simulink model "ibob_phased_array_2k"  (Simulink 7.1)
settings: Solver=ode45  StartTime=0.0  StopTime=70  RelTol=1e-3
undefined symbols (not defined in the file or in its folder): iBOB
libraries: xbsIndex_r4 x1407, xps_library x46, cfa_library x16, casper_library_sources x8, casper_library_misc x4
(part 3 of 18)

== system ibob_phased_array_2k/gain_calib3 ==
  gain : Inport  OutDataType=sfix(16)  OutScaling=2^0
  in : Inport  Port=2  OutDataType=sfix(16)  OutScaling=2^0
  Concat : xbsIndex_r4/Concat  num_inputs=4  dbl_ovrd=off  block_type=concat
      settings: block_version=10.1.3
  Delay{1..4} (4 alike) : xbsIndex_r4/Delay  en=off  latency=1  dbl_ovrd=off  reg_retiming=off  block_type=delay
  Mult{,1..3} (4 alike) : xbsIndex_r4/Mult  precision=Full  arith_type="Signed  (2's comp)"  n_bits=8  bin_pt=2  quantization=Truncate  overflow=Wrap  en=off  latency=7  dbl_ovrd=off  use_behavioral_HDL=off  use_embedded=on  opt=Speed  optimum_pipeline=off  pipeline=on  use_rpm=on  placement_style=Rectangular shape  block_type=mult
      settings: infoedit=Hardware notes: To use the internal pipeline stage of the dedicated multiplier you must select 'Pipeline for maximum performance'.  xl_area=[0, 0, 0, 0, 0, 0, 0]  block_version=10.1.3
  Reinterpret{,1..3} (4 alike) : xbsIndex_r4/Reinterpret  force_arith_type=on  arith_type=Unsigned  force_bin_pt=on  bin_pt=0  block_type=reinterpret
      settings: infoedit="Changes signal type without altering the binary representation.   You can changed the signal between signed and unsigned, and relocate the binary point.<P><P>Hardware notes: In hardware this block costs nothing.<P><P>Example:  Suppose the input is 6 bits wide, signed, with 2 fractional bits, and the output is forced to unsigned with 0 fractional bits.  Then an input of -2.0 (1110.00 in binary 2's complement) becomes an output of 56 (111000 in binary)."  block_version=10.1.3
  Reinterpret4 : xbsIndex_r4/Reinterpret  force_arith_type=on  arith_type=Unsigned  force_bin_pt=on  bin_pt=7  block_type=reinterpret
      settings: infoedit="Changes signal type without altering the binary representation.   You can changed the signal between signed and unsigned, and relocate the binary point.<P><P>Hardware notes: In hardware this block costs nothing.<P><P>Example:  Suppose the input is 6 bits wide, signed, with 2 fractional bits, and the output is forced to unsigned with 0 fractional bits.  Then an input of -2.0 (1110.00 in binary 2's complement) becomes an output of 56 (111000 in binary)."  block_version=10.1.3
  Slice2 : xbsIndex_r4/Slice  nbits=8  boolean_output=off  mode=Lower Bit Location + Width  bit1=0  base1=MSB of Input  bit0=0  base0=LSB of Input  dbl_ovrd=off  block_type=slice
      settings: infoedit="Extracts a given range of bits from each input sample and presents it at the output.  The output type is ordinarily unsigned with binary point at zero, but can be Boolean when the slice is one bit wide.<P><P>Hardware notes: In hardware this block costs nothing."  block_version=10.1.3
  convert1 : Subsystem  AncestorBlock=casper_library_misc/convert  mask(convert){bin_pt_in=7, n_bits_out=8, bin_pt_out=0, quantization=Round  (unbiased: +/- Inf), overflow=Saturate, latency=1}
      mask prompts: bin_pt_in "Binary Point In"; n_bits_out "Bit Width Out"; bin_pt_out "Binary Point Out"
      mask help:
      | Convert input value to the specified bit width and precision.
      |
      | Does not support upscaling number of fractional bits (eg 8_5 to 8_4 is ok, but not 8_4 to 8_5).
      mask init: same as ibob_phased_array_2k/gain_calib0/convert1
      settings: AttributesFormatString=|
      | N_7 ==> 8_0
      | round inf, saturate
      | latency = 1
      mask Help:
      | <pre>
      | Description::
      | 
      | Outputs converted version of the input.
      | 
      | Mask Parameters::
      | 
      | Binary Point In (bin_pt_in): Specifies the binary point location in the input.
      | 
      | Bit Width Out (n_bits_out): Specifies the width of the output.
      | 
      | Binary Point Out (bin_pt_out): Specifies the binary point location in the output.
      | 
      | Quantization (quantization): Specifies quantization handling.
      | 
      | Overflow (overflow): Specifies overflow handling.
      | 
      | Latency (latency): Specifies the latency of the underlying adder block, which is the overall
      | latency of this block as well.
      | </pre>
      mask StyleString: edit,edit,edit,popup(Truncate|Round  (unbiased: +/- Inf)|Round  (unbiased: Even Values)|Round  (unbiased: Zero)|Round  (unbiased: Odd Values)|Round  (biased: Up)|Round  (biased: Down)),popup(Wrap|Saturate|Error),edit
  convert2 : Subsystem  AncestorBlock=casper_library_misc/convert  mask(convert){bin_pt_in=7, n_bits_out=8, bin_pt_out=0, quantization=Round  (unbiased: +/- Inf), overflow=Saturate, latency=1}
      mask prompts: bin_pt_in "Binary Point In"; n_bits_out "Bit Width Out"; bin_pt_out "Binary Point Out"
      mask help:
      | Convert input value to the specified bit width and precision.
      |
      | Does not support upscaling number of fractional bits (eg 8_5 to 8_4 is ok, but not 8_4 to 8_5).
      mask init: same as ibob_phased_array_2k/gain_calib0/convert1
      settings: AttributesFormatString=|
      | N_7 ==> 8_0
      | round inf, saturate
      | latency = 1
      mask Help:
      | <pre>
      | Description::
      | 
      | Outputs converted version of the input.
      | 
      | Mask Parameters::
      | 
      | Binary Point In (bin_pt_in): Specifies the binary point location in the input.
      | 
      | Bit Width Out (n_bits_out): Specifies the width of the output.
      | 
      | Binary Point Out (bin_pt_out): Specifies the binary point location in the output.
      | 
      | Quantization (quantization): Specifies quantization handling.
      | 
      | Overflow (overflow): Specifies overflow handling.
      | 
      | Latency (latency): Specifies the latency of the underlying adder block, which is the overall
      | latency of this block as well.
      | </pre>
      mask StyleString: edit,edit,edit,popup(Truncate|Round  (unbiased: +/- Inf)|Round  (unbiased: Even Values)|Round  (unbiased: Zero)|Round  (unbiased: Odd Values)|Round  (biased: Up)|Round  (biased: Down)),popup(Wrap|Saturate|Error),edit
  convert3 : Subsystem  AncestorBlock=casper_library_misc/convert  mask(convert){bin_pt_in=7, n_bits_out=8, bin_pt_out=0, quantization=Round  (unbiased: +/- Inf), overflow=Saturate, latency=1}
      mask prompts: bin_pt_in "Binary Point In"; n_bits_out "Bit Width Out"; bin_pt_out "Binary Point Out"
      mask help:
      | Convert input value to the specified bit width and precision.
      |
      | Does not support upscaling number of fractional bits (eg 8_5 to 8_4 is ok, but not 8_4 to 8_5).
      mask init: same as ibob_phased_array_2k/gain_calib0/convert1
      settings: AttributesFormatString=|
      | N_7 ==> 8_0
      | round inf, saturate
      | latency = 1
      mask Help:
      | <pre>
      | Description::
      | 
      | Outputs converted version of the input.
      | 
      | Mask Parameters::
      | 
      | Binary Point In (bin_pt_in): Specifies the binary point location in the input.
      | 
      | Bit Width Out (n_bits_out): Specifies the width of the output.
      | 
      | Binary Point Out (bin_pt_out): Specifies the binary point location in the output.
      | 
      | Quantization (quantization): Specifies quantization handling.
      | 
      | Overflow (overflow): Specifies overflow handling.
      | 
      | Latency (latency): Specifies the latency of the underlying adder block, which is the overall
      | latency of this block as well.
      | </pre>
      mask StyleString: edit,edit,edit,popup(Truncate|Round  (unbiased: +/- Inf)|Round  (unbiased: Even Values)|Round  (unbiased: Zero)|Round  (unbiased: Odd Values)|Round  (biased: Up)|Round  (biased: Down)),popup(Wrap|Saturate|Error),edit
  convert4 : Subsystem  AncestorBlock=casper_library_misc/convert  mask(convert){bin_pt_in=7, n_bits_out=8, bin_pt_out=0, quantization=Round  (unbiased: +/- Inf), overflow=Saturate, latency=1}
      mask prompts: bin_pt_in "Binary Point In"; n_bits_out "Bit Width Out"; bin_pt_out "Binary Point Out"
      mask help:
      | Convert input value to the specified bit width and precision.
      |
      | Does not support upscaling number of fractional bits (eg 8_5 to 8_4 is ok, but not 8_4 to 8_5).
      mask init: same as ibob_phased_array_2k/gain_calib0/convert1
      settings: AttributesFormatString=|
      | N_7 ==> 8_0
      | round inf, saturate
      | latency = 1
      mask Help:
      | <pre>
      | Description::
      | 
      | Outputs converted version of the input.
      | 
      | Mask Parameters::
      | 
      | Binary Point In (bin_pt_in): Specifies the binary point location in the input.
      | 
      | Bit Width Out (n_bits_out): Specifies the width of the output.
      | 
      | Binary Point Out (bin_pt_out): Specifies the binary point location in the output.
      | 
      | Quantization (quantization): Specifies quantization handling.
      | 
      | Overflow (overflow): Specifies overflow handling.
      | 
      | Latency (latency): Specifies the latency of the underlying adder block, which is the overall
      | latency of this block as well.
      | </pre>
      mask StyleString: edit,edit,edit,popup(Truncate|Round  (unbiased: +/- Inf)|Round  (unbiased: Even Values)|Round  (unbiased: Zero)|Round  (unbiased: Odd Values)|Round  (biased: Up)|Round  (biased: Down)),popup(Wrap|Saturate|Error),edit
  slice2 : Subsystem
  out : Outport  OutDataType=sfix(16)  OutScaling=2^0
  wires:
  in/1 -> slice2/1(in)
  slice2/1(out0) -> Mult/1
  slice2/2(out1) -> Mult1/1
  slice2/3(out2) -> Mult2/1
  slice2/4(out3) -> Mult3/1
  gain/1 -> Slice2/1
  Mult/1 -> Delay1/1
  Mult1/1 -> Delay2/1
  Mult2/1 -> Delay3/1
  Mult3/1 -> Delay4/1
  Concat/1 -> out/1
  convert4/1(out) -> Reinterpret3/1
  convert3/1(out) -> Reinterpret2/1
  convert1/1(out) -> Reinterpret1/1
  convert2/1(out) -> Reinterpret/1
  Slice2/1 -> Reinterpret4/1
  Reinterpret/1 -> Concat/1
  Reinterpret1/1 -> Concat/2
  Reinterpret2/1 -> Concat/3
  Reinterpret3/1 -> Concat/4
  Reinterpret4/1 -> Mult3/2, Mult2/2, Mult1/2, Mult/2
  Delay1/1 -> convert2/1(in)
  Delay2/1 -> convert1/1(in)
  Delay3/1 -> convert3/1(in)
  Delay4/1 -> convert4/1(in)

== system ibob_phased_array_2k/hb_sync ==
  note: SOWF = Start Of Walsh Frame
      | HB = Heart-Beat (roughly 100pps)
  Step : Step  Time=200  Before=1  After=0  SampleTime=1
  Terminator : Terminator
  arm_sowf : xps_library/software register  Tag=xps:sw_reg  SystemSampleTime=-1  io_dir=From Processor  arith_type=Unsigned  bitwidth=32  bin_pt=0  sample_period=1  gw_name=ibob_phased_array_2k_hb_sync_arm_sowf_user_data_out
      link override dbe_xaui_corr_onepps_sync_arm1pps_user_data_out: arith_type=Unsigned  n_bits=32  bin_pt=0  period=1
      link override dbe_xaui_onepps_sync_arm1pps_user_data_out: arith_type=Unsigned  n_bits=32  bin_pt=0  period=1
      link override ibob_phased_array_2k_hb_sync_arm_sowf_user_data_out: arith_type=Unsigned  n_bits=32  bin_pt=0  period=1
      link override ibob_phased_array_2k_onepps_sync_arm1pps_user_data_out: arith_type=Unsigned  n_bits=32  bin_pt=0  period=1
      link override vlbipfb2_m3_ibob_onepps_sync_arm1pps_user_data_out: arith_type=Unsigned  n_bits=32  bin_pt=0  period=1
      link override vlbipfb2_m3_roach_onepps_sync_arm1pps_user_data_out: arith_type=Unsigned  n_bits=32  bin_pt=0  period=1
  armshake : Subsystem
  armsowf_ack : xps_library/software register  Tag=xps:sw_reg  SystemSampleTime=-1  io_dir=To Processor  arith_type=Unsigned  bitwidth=32  bin_pt=0  sample_period=1  gw_name=ibob_phased_array_2k_hb_sync_armsowf_ack_user_data_in
      link override convert: arith_type=Unsigned  n_bits=32  bin_pt=0
  hb_gen : Subsystem  mask{samples=2581110}
      mask prompts: samples "Period:"
  sowf_gen : Subsystem  mask{samples=2581110*32}
      mask prompts: samples "Period:"
  tag scope: int_hb=global, int_sowf=global
  wires:
  [sync0] -> armshake/1(ext_sowf)
  armsowf_ack/1 -> Terminator/1
  armshake/2(arm_ack) -> armsowf_ack/1
  armshake/1(rst_sowf) -> sowf_gen/1(rst), hb_gen/1(rst)
  Step/1 -> arm_sowf/1
  arm_sowf/1 -> armshake/2(ext_armsowf)
  sowf_gen/1(1pps) -> [int_sowf]
  hb_gen/1(1pps) -> [int_hb]

== system ibob_phased_array_2k/noise ==
  note: These are the "seed" and "arm" control registers
      | and the slicing of the "insel" register
      | for thenoise generators, which
      | live in the input_mux block.
  note: Arming is done using rising edge of
      | (one bit of) one nybble per input...
      |
      | 0x0001 = Arm input 0
      | 0x0010 = Arm input 1
      | 0x0100 = Arm input 2
      | 0x1000 = Arm input 3
  note: Input selection uses one bit per demux path per input.
      | 0 == Use ADC; 1 == Use noise source.
      |
      | 0x0000 = Select ADC for all demux paths of all inputs
      | 0x0001 = Select noise source for demux path 0 of input0, select ADC  for all other demux paths
      | 0x000F = Seelct noise source for all demux paths of input 0, select ADC for all other inputs
      | 0xFFFF = Select noise source for all demux paths of all inputs
      | 0xF000 = Select noise source for all demux paths of input 3, select ADC for all other inputs
      | 0xC000 = Select noise source for demux paths 2 and 3 of input 3, select ADC for all other inputs
  BitBasher : xbsIndex_r4/BitBasher  bitexpr=|  display_expr=off  sr_1=1  arith_type1=Unsigned  bin_pt1=0  sr_2=2  arith_type2=Unsigned  bin_pt2=0  sr_3=3  arith_type3=Unsigned  bin_pt3=0  sr_4=4  arith_type4=Unsigned  bin_pt4=0  dbl_ovrd=off  block_type=bitbasher
      | <html><head><meta name="qrichtext" content="1" /><style type="text/css">
      | p, li { white-space: pre-wrap; }
      | </style></head><body style=" font-family:'MS Shell Dlg 2'; font-size:8.25pt; font-weight:400; font-style:normal;">
      | <p style=" margin-top:12px; margin-bottom:12px; margin-left:0px; margin-right:0px; -qt-block-indent:0; text-indent:0px; font-family:'MS Shell Dlg'; font-size:8pt;">arm0={arm[0]}<br />arm1={arm[4]}<br />arm2={arm[8]}<br />arm3={arm[12]}<br /></p></body></html>
      settings: block_version=10.1.3
  BitBasher1 : xbsIndex_r4/BitBasher  bitexpr=|  display_expr=off  sr_1=1  arith_type1=Unsigned  bin_pt1=0  sr_2=2  arith_type2=Unsigned  bin_pt2=0  sr_3=3  arith_type3=Unsigned  bin_pt3=0  sr_4=4  arith_type4=Unsigned  bin_pt4=0  dbl_ovrd=off  block_type=bitbasher
      | <html><head><meta name="qrichtext" content="1" /><style type="text/css">
      | p, li { white-space: pre-wrap; }
      | </style></head><body style=" font-family:'MS Shell Dlg 2'; font-size:8.25pt; font-weight:400; font-style:normal;">
      | <p style=" margin-top:12px; margin-bottom:12px; margin-left:0px; margin-right:0px; -qt-block-indent:0; text-indent:0px; font-family:'MS Shell Dlg'; font-size:8pt;">insel0={insel[3:0]}<br />insel1={insel[7:4]}<br />insel2={insel[11:8]}<br />insel3={insel[15:12]}<br /></p></body></html>
      settings: block_version=10.1.3
  Constant10 : Constant  Value=0
  arm : xps_library/software register  Tag=xps:sw_reg  SystemSampleTime=-1  io_dir=From Processor  arith_type=Unsigned  bitwidth=32  bin_pt=0  sample_period=1  gw_name=ibob_phased_array_2k_noise_arm_user_data_out
      link override dbe_adc_single_noise_arm_user_data_out: arith_type=Unsigned  n_bits=32  bin_pt=0  period=1
      link override dbe_adc_single_shiftctrl_reg_user_data_out: arith_type=Unsigned  n_bits=32  bin_pt=0  period=1
      link override ibob_phased_array_2k_noise_arm_user_data_out: arith_type=Unsigned  n_bits=32  bin_pt=0  period=1
      link override vlbipfb2_m3_ibob_shiftctrl_reg_user_data_out: arith_type=Unsigned  n_bits=32  bin_pt=0  period=1
      link override vlbipfb2_m3_roach_shiftctrl_reg_user_data_out: arith_type=Unsigned  n_bits=32  bin_pt=0  period=1
  seed : Subsystem
  tag scope: insel0=global, insel1=global, insel2=global, insel3=global, wgn_arm0=global, wgn_arm1=global, wgn_arm2=global, wgn_arm3=global
  wires:
  arm/1 -> BitBasher/1
  Constant10/1 -> arm/1
  BitBasher/1 -> [wgn_arm0]
  BitBasher/2 -> [wgn_arm1]
  BitBasher/3 -> [wgn_arm2]
  BitBasher/4 -> [wgn_arm3]
  BitBasher1/1 -> [insel0]
  BitBasher1/2 -> [insel1]
  BitBasher1/3 -> [insel2]
  BitBasher1/4 -> [insel3]
  [insel] -> BitBasher1/1

== system ibob_phased_array_2k/onepps_sync ==
  Mux3 : xbsIndex_r4/Mux  inputs=2  en=off  latency=0  precision=Full  arith_type="Signed  (2's comp)"  n_bits=8  bin_pt=2  quantization=Truncate  overflow=Wrap  dbl_ovrd=off  block_type=mux
      settings: xl_area=[0, 0, 0, 0, 0, 0, 0]
  Step : Step  Time=200  Before=1  After=0  SampleTime=1
  Terminator : Terminator
  arm1pps : xps_library/software register  Tag=xps:sw_reg  SystemSampleTime=-1  io_dir=From Processor  arith_type=Unsigned  bitwidth=32  bin_pt=0  sample_period=1  gw_name=ibob_phased_array_2k_onepps_sync_arm1pps_user_data_out
      link override dbe_xaui_corr_onepps_sync_arm1pps_user_data_out: arith_type=Unsigned  n_bits=32  bin_pt=0  period=1
      link override dbe_xaui_onepps_sync_arm1pps_user_data_out: arith_type=Unsigned  n_bits=32  bin_pt=0  period=1
      link override ibob_phased_array_2k_onepps_sync_arm1pps_user_data_out: arith_type=Unsigned  n_bits=32  bin_pt=0  period=1
      link override vlbipfb2_m3_ibob_onepps_sync_arm1pps_user_data_out: arith_type=Unsigned  n_bits=32  bin_pt=0  period=1
      link override vlbipfb2_m3_roach_onepps_sync_arm1pps_user_data_out: arith_type=Unsigned  n_bits=32  bin_pt=0  period=1
  arm1pps_ack : xps_library/software register  Tag=xps:sw_reg  SystemSampleTime=-1  io_dir=To Processor  arith_type=Unsigned  bitwidth=32  bin_pt=0  sample_period=1  gw_name=ibob_phased_array_2k_onepps_sync_arm1pps_ack_user_data_in
      link override convert: arith_type=Unsigned  n_bits=32  bin_pt=0
  armshake : Subsystem
  int_1024pps_gen : Subsystem
  int_1pps_gen : Subsystem
  lsb : xbsIndex_r4/Slice  nbits=1  boolean_output=off  mode=Lower Bit Location + Width  bit1=0  base1=MSB of Input  bit0=0  base0=LSB of Input  dbl_ovrd=off  block_type=slice
      settings: infoedit="Extracts a given range of bits from each input sample and presents it at the output.  The output type is ordinarily unsigned with binary point at zero, but can be Boolean when the slice is one bit wide.<P><P>Hardware notes: In hardware this block costs nothing."  block_version=10.1.3
  tag scope: int_1024pps=global, int_1pps=global
  wires:
  int_1pps_gen/1(1pps) -> [int_1pps]
  Mux3/1 -> armshake/1(ext_1pps)
  arm1pps/1 -> armshake/2(ext_arm1pps)
  Step/1 -> arm1pps/1
  armshake/1(rst_1pps) -> int_1pps_gen/1(rst), int_1024pps_gen/1(rst)
  armshake/2(arm_ack) -> arm1pps_ack/1
  arm1pps_ack/1 -> Terminator/1
  [ppssel] -> lsb/1
  [sync0] -> Mux3/2
  [sync1] -> Mux3/3
  lsb/1 -> Mux3/1
  int_1024pps_gen/1(1pps) -> [int_1024pps]

== system ibob_phased_array_2k/quant ==
  note: 4 cycles latency from iN to qN
  i0 : Inport
  i1 : Inport  Port=2
  i2 : Inport  Port=3
  i3 : Inport  Port=4
  BitBasher : xbsIndex_r4/BitBasher  bitexpr=|  display_expr=off  sr_1=1  arith_type1="Signed  (2's comp)"  bin_pt1=0  sr_2=2  arith_type2="Signed  (2's comp)"  bin_pt2=0  sr_3=3  arith_type3="Signed  (2's comp)"  bin_pt3=0  sr_4=4  arith_type4="Signed  (2's comp)"  bin_pt4=0  dbl_ovrd=off  block_type=bitbasher
      | <html><head><meta name="qrichtext" content="1" /><style type="text/css">
      | p, li { white-space: pre-wrap; }
      | </style></head><body style=" font-family:'MS Shell Dlg 2'; font-size:8.25pt; font-weight:400; font-style:normal;">
      | <p style=" margin-top:0px; margin-bottom:0px; margin-left:0px; margin-right:0px; -qt-block-indent:0; text-indent:0px; font-size:8pt;">in0={in[31:24]}<br />in1={in[23:16]}<br />in2={in[15:8]}<br />in3={in[7:0]}<br /></p></body></html>
      settings: block_version=10.1.3
  BitBasher1 : xbsIndex_r4/BitBasher  bitexpr=|  display_expr=off  sr_1=1  arith_type1="Signed  (2's comp)"  bin_pt1=0  sr_2=2  arith_type2="Signed  (2's comp)"  bin_pt2=0  sr_3=3  arith_type3="Signed  (2's comp)"  bin_pt3=0  sr_4=4  arith_type4="Signed  (2's comp)"  bin_pt4=0  dbl_ovrd=off  block_type=bitbasher
      | <html><head><meta name="qrichtext" content="1" /><style type="text/css">
      | p, li { white-space: pre-wrap; }
      | </style></head><body style=" font-family:'MS Shell Dlg 2'; font-size:8.25pt; font-weight:400; font-style:normal;">
      | <p style=" margin-top:0px; margin-bottom:0px; margin-left:0px; margin-right:0px; -qt-block-indent:0; text-indent:0px; font-size:8pt;">in0={in[31:24]}<br />in1={in[23:16]}<br />in2={in[15:8]}<br />in3={in[7:0]}<br /></p></body></html>
      settings: block_version=10.1.3
  BitBasher2 : xbsIndex_r4/BitBasher  bitexpr=|  display_expr=off  sr_1=1  arith_type1="Signed  (2's comp)"  bin_pt1=0  sr_2=2  arith_type2="Signed  (2's comp)"  bin_pt2=0  sr_3=3  arith_type3="Signed  (2's comp)"  bin_pt3=0  sr_4=4  arith_type4="Signed  (2's comp)"  bin_pt4=0  dbl_ovrd=off  block_type=bitbasher
      | <html><head><meta name="qrichtext" content="1" /><style type="text/css">
      | p, li { white-space: pre-wrap; }
      | </style></head><body style=" font-family:'MS Shell Dlg 2'; font-size:8.25pt; font-weight:400; font-style:normal;">
      | <p style=" margin-top:0px; margin-bottom:0px; margin-left:0px; margin-right:0px; -qt-block-indent:0; text-indent:0px; font-size:8pt;">in0={in[31:24]}<br />in1={in[23:16]}<br />in2={in[15:8]}<br />in3={in[7:0]}<br /></p></body></html>
      settings: block_version=10.1.3
  BitBasher3 : xbsIndex_r4/BitBasher  bitexpr=|  display_expr=off  sr_1=1  arith_type1="Signed  (2's comp)"  bin_pt1=0  sr_2=2  arith_type2="Signed  (2's comp)"  bin_pt2=0  sr_3=3  arith_type3="Signed  (2's comp)"  bin_pt3=0  sr_4=4  arith_type4="Signed  (2's comp)"  bin_pt4=0  dbl_ovrd=off  block_type=bitbasher
      | <html><head><meta name="qrichtext" content="1" /><style type="text/css">
      | p, li { white-space: pre-wrap; }
      | </style></head><body style=" font-family:'MS Shell Dlg 2'; font-size:8.25pt; font-weight:400; font-style:normal;">
      | <p style=" margin-top:0px; margin-bottom:0px; margin-left:0px; margin-right:0px; -qt-block-indent:0; text-indent:0px; font-size:8pt;">in0={in[31:24]}<br />in1={in[23:16]}<br />in2={in[15:8]}<br />in3={in[7:0]}<br /></p></body></html>
      settings: block_version=10.1.3
  BitBasher4 : xbsIndex_r4/BitBasher  bitexpr=|  display_expr=off  sr_1=1  arith_type1=Unsigned  bin_pt1=0  sr_2=2  arith_type2="Signed  (2's comp)"  bin_pt2=7  sr_3=3  arith_type3="Signed  (2's comp)"  bin_pt3=7  sr_4=4  arith_type4="Signed  (2's comp)"  bin_pt4=7  dbl_ovrd=off  block_type=bitbasher
      | <html><head><meta name="qrichtext" content="1" /><style type="text/css">
      | p, li { white-space: pre-wrap; }
      | </style></head><body style=" font-family:'MS Shell Dlg 2'; font-size:8.25pt; font-weight:400; font-style:normal;">
      | <p style=" margin-top:0px; margin-bottom:0px; margin-left:0px; margin-right:0px; -qt-block-indent:0; text-indent:0px; font-size:8pt;">out={in0,in1,in2,in3}</p></body></html>
      settings: block_version=10.1.3
  BitBasher5 : xbsIndex_r4/BitBasher  bitexpr=|  display_expr=off  sr_1=1  arith_type1=Unsigned  bin_pt1=0  sr_2=2  arith_type2="Signed  (2's comp)"  bin_pt2=7  sr_3=3  arith_type3="Signed  (2's comp)"  bin_pt3=7  sr_4=4  arith_type4="Signed  (2's comp)"  bin_pt4=7  dbl_ovrd=off  block_type=bitbasher
      | <html><head><meta name="qrichtext" content="1" /><style type="text/css">
      | p, li { white-space: pre-wrap; }
      | </style></head><body style=" font-family:'MS Shell Dlg 2'; font-size:8.25pt; font-weight:400; font-style:normal;">
      | <p style=" margin-top:0px; margin-bottom:0px; margin-left:0px; margin-right:0px; -qt-block-indent:0; text-indent:0px; font-size:8pt;">out={in0,in1,in2,in3}</p></body></html>
      settings: block_version=10.1.3
  BitBasher6 : xbsIndex_r4/BitBasher  bitexpr=|  display_expr=off  sr_1=1  arith_type1=Unsigned  bin_pt1=0  sr_2=2  arith_type2="Signed  (2's comp)"  bin_pt2=7  sr_3=3  arith_type3="Signed  (2's comp)"  bin_pt3=7  sr_4=4  arith_type4="Signed  (2's comp)"  bin_pt4=7  dbl_ovrd=off  block_type=bitbasher
      | <html><head><meta name="qrichtext" content="1" /><style type="text/css">
      | p, li { white-space: pre-wrap; }
      | </style></head><body style=" font-family:'MS Shell Dlg 2'; font-size:8.25pt; font-weight:400; font-style:normal;">
      | <p style=" margin-top:0px; margin-bottom:0px; margin-left:0px; margin-right:0px; -qt-block-indent:0; text-indent:0px; font-size:8pt;">out={in0,in1,in2,in3}</p></body></html>
      settings: block_version=10.1.3
  BitBasher7 : xbsIndex_r4/BitBasher  bitexpr=|  display_expr=off  sr_1=1  arith_type1=Unsigned  bin_pt1=0  sr_2=2  arith_type2="Signed  (2's comp)"  bin_pt2=7  sr_3=3  arith_type3="Signed  (2's comp)"  bin_pt3=7  sr_4=4  arith_type4="Signed  (2's comp)"  bin_pt4=7  dbl_ovrd=off  block_type=bitbasher
      | <html><head><meta name="qrichtext" content="1" /><style type="text/css">
      | p, li { white-space: pre-wrap; }
      | </style></head><body style=" font-family:'MS Shell Dlg 2'; font-size:8.25pt; font-weight:400; font-style:normal;">
      | <p style=" margin-top:0px; margin-bottom:0px; margin-left:0px; margin-right:0px; -qt-block-indent:0; text-indent:0px; font-size:8pt;">out={in0,in1,in2,in3}</p></body></html>
      settings: block_version=10.1.3
  Constant{1..3,23} (4 alike) : Constant  OutDataType=sfix(16)  OutScaling=2^0
  Slice{1..4} (4 alike) : xbsIndex_r4/Slice  nbits=7  boolean_output=off  mode=Lower Bit Location + Width  bit1=0  base1=MSB of Input  bit0=0  base0=LSB of Input  dbl_ovrd=off  block_type=slice
      settings: infoedit="Extracts a given range of bits from each input sample and presents it at the output.  The output type is ordinarily unsigned with binary point at zero, but can be Boolean when the slice is one bit wide.<P><P>Hardware notes: In hardware this block costs nothing."  block_version=10.1.3
  quant0 : Subsystem
  quant1 : Subsystem
  quant2 : Subsystem
  quant3 : Subsystem
  thresh0 : xps_library/software register  Tag=xps:sw_reg  SystemSampleTime=-1  io_dir=From Processor  arith_type=Unsigned  bitwidth=32  bin_pt=0  sample_period=1  gw_name=ibob_phased_array_2k_quant_thresh0_user_data_out
      link override ibob_phased_array_2k_quant_thresh0_user_data_out: arith_type=Unsigned  n_bits=32  bin_pt=0  period=1
      link override ibob_phased_array_2k_thresh0_user_data_out: arith_type=Unsigned  n_bits=32  bin_pt=0  period=1
  thresh1 : xps_library/software register  Tag=xps:sw_reg  SystemSampleTime=-1  io_dir=From Processor  arith_type=Unsigned  bitwidth=32  bin_pt=0  sample_period=1  gw_name=ibob_phased_array_2k_quant_thresh1_user_data_out
      link override ibob_phased_array_2k_quant_thresh1_user_data_out: arith_type=Unsigned  n_bits=32  bin_pt=0  period=1
      link override ibob_phased_array_2k_thresh0_user_data_out: arith_type=Unsigned  n_bits=32  bin_pt=0  period=1
  thresh2 : xps_library/software register  Tag=xps:sw_reg  SystemSampleTime=-1  io_dir=From Processor  arith_type=Unsigned  bitwidth=32  bin_pt=0  sample_period=1  gw_name=ibob_phased_array_2k_quant_thresh2_user_data_out
      link override ibob_phased_array_2k_quant_thresh2_user_data_out: arith_type=Unsigned  n_bits=32  bin_pt=0  period=1
      link override ibob_phased_array_2k_thresh0_user_data_out: arith_type=Unsigned  n_bits=32  bin_pt=0  period=1
  thresh3 : xps_library/software register  Tag=xps:sw_reg  SystemSampleTime=-1  io_dir=From Processor  arith_type=Unsigned  bitwidth=32  bin_pt=0  sample_period=1  gw_name=ibob_phased_array_2k_quant_thresh3_user_data_out
      link override ibob_phased_array_2k_quant_thresh3_user_data_out: arith_type=Unsigned  n_bits=32  bin_pt=0  period=1
      link override ibob_phased_array_2k_thresh0_user_data_out: arith_type=Unsigned  n_bits=32  bin_pt=0  period=1
  q0 : Outport  OutDataType=sfix(16)  OutScaling=2^0
  q1 : Outport  Port=2  OutDataType=sfix(16)  OutScaling=2^0
  q2 : Outport  Port=3  OutDataType=sfix(16)  OutScaling=2^0
  q3 : Outport  Port=4  OutDataType=sfix(16)  OutScaling=2^0
  wires:
  thresh0/1 -> Slice3/1
  Constant23/1 -> thresh0/1
  Slice3/1 -> quant0/1(thresh)
  i0/1 -> BitBasher/1
  BitBasher/1 -> quant0/2(i0)
  BitBasher/2 -> quant0/3(i1)
  BitBasher/3 -> quant0/4(i2)
  BitBasher/4 -> quant0/5(i3)
  thresh1/1 -> Slice1/1
  Constant1/1 -> thresh1/1
  Slice1/1 -> quant1/1(thresh)
  i1/1 -> BitBasher1/1
  BitBasher1/1 -> quant1/2(i0)
  BitBasher1/2 -> quant1/3(i1)
  BitBasher1/3 -> quant1/4(i2)
  BitBasher1/4 -> quant1/5(i3)
  thresh2/1 -> Slice2/1
  Constant2/1 -> thresh2/1
  Slice2/1 -> quant2/1(thresh)
  i2/1 -> BitBasher2/1
  BitBasher2/1 -> quant2/2(i0)
  BitBasher2/2 -> quant2/3(i1)
  BitBasher2/3 -> quant2/4(i2)
  BitBasher2/4 -> quant2/5(i3)
  thresh3/1 -> Slice4/1
  Constant3/1 -> thresh3/1
  Slice4/1 -> quant3/1(thresh)
  i3/1 -> BitBasher3/1
  BitBasher3/1 -> quant3/2(i0)
  BitBasher3/2 -> quant3/3(i1)
  BitBasher3/3 -> quant3/4(i2)
  BitBasher3/4 -> quant3/5(i3)
  BitBasher4/1 -> q0/1
  quant0/1(q0) -> BitBasher4/1
  quant0/2(q1) -> BitBasher4/2
  quant0/3(q2) -> BitBasher4/3
  quant0/4(q3) -> BitBasher4/4
  BitBasher5/1 -> q1/1
  quant1/1(q0) -> BitBasher5/1
  quant1/2(q1) -> BitBasher5/2
  quant1/3(q2) -> BitBasher5/3
  quant1/4(q3) -> BitBasher5/4
  BitBasher6/1 -> q2/1
  quant2/1(q0) -> BitBasher6/1
  quant2/2(q1) -> BitBasher6/2
  quant2/3(q2) -> BitBasher6/3
  quant2/4(q3) -> BitBasher6/4
  BitBasher7/1 -> q3/1
  quant3/1(q0) -> BitBasher7/1
  quant3/2(q1) -> BitBasher7/2
  quant3/3(q2) -> BitBasher7/3
  quant3/4(q3) -> BitBasher7/4

== system ibob_phased_array_2k/sync_demux2 ==
  note: We want to send 7 signals over OOB (3 syncs + 4 walsh states),
      | so we need to do special demux here and special mux on other
      | side.  We want to send 8 bit OOB and 32 bit data.  This mean that
      | a 1 cycle sync0 signal would be missed whenever it occurs the
      | cycle after int_1024pps goes high.  To avoid this, we stretch out
      | the sync0 signal by one cycle.  We also delay the sync and walsh
      | so that they will be sent along with the data samples that reflect
      | the wlash state being transmitted.
      |
      | walsh select latency = 5 cycles
      | phase switch latency = 21 cycles
      | 2-bit quantize latency = 4 cycles
  note: ___
      | 1024pps __/   \______________________
      |           | A       B
      |         __ __________________________
      | w[3:0]  __X__________________________
      |           | A       B
      |                ___
      | sync0   ______/   \__________________
      |           |
      |                _______
      | sync0s  ______/       \_______________
      |           |         B
      |         __ ___ ___ ___ ___ ___ ___ __
      | d[31:0] __X___X___X___X___X___X___X__
      |           | 0   1
      |         __ ___     ___     ___     __
      | valid   __X___X___/   \___/   \___/
      |           |         !       !
      |        _______ _______ _______ ______
      | oob    _______X_______X_______X______
      |           |       A !     B !
      |         ______ _______ _______ ______
      | first   ______X_______X_______X______
      |           |       0 !     2 !
      |         __ _______ _______ _______ __
      | second  __X_______X_______X_______X__
      |           |         ! 1     ! 3
  din : Inport
  BitBasher1 : xbsIndex_r4/BitBasher  bitexpr=|  display_expr=off  sr_1=1  arith_type1=Unsigned  bin_pt1=0  sr_2=2  arith_type2=Unsigned  bin_pt2=0  sr_3=3  arith_type3=Unsigned  bin_pt3=0  sr_4=4  arith_type4=Unsigned  bin_pt4=0  dbl_ovrd=off  block_type=bitbasher
      | <html><head><meta name="qrichtext" content="1" /><style type="text/css">
      | p, li { white-space: pre-wrap; }
      | </style></head><body style=" font-family:'MS Shell Dlg 2'; font-size:8.25pt; font-weight:400; font-style:normal;">
      | <p style=" margin-top:12px; margin-bottom:12px; margin-left:0px; margin-right:0px; -qt-block-indent:0; text-indent:0px; font-family:'MS Shell Dlg'; font-size:8pt;">oob={1'b0,sync0,pps1,pps1024,w3[0],w2[0],w1[0],w0[0]}</p></body></html>
      settings: block_version=10.1.3
  Concat3 : xbsIndex_r4/Concat  num_inputs=2  dbl_ovrd=off  block_type=concat
      settings: block_version=10.1.3
  Counter : xbsIndex_r4/Counter  cnt_type=Free Running  cnt_to=Inf  operation=Up  start_count=0  cnt_by_val=1  arith_type=Unsigned  n_bits=1  bin_pt=0  load_pin=off  rst=on  en=on  explicit_period=on  period=1  dbl_ovrd=off  use_behavioral_HDL=off  use_rpm=off  implementation=Fabric  block_type=counter
  Delay{1,3..8} (7 alike) : xbsIndex_r4/Delay  en=off  latency=walsh_delay+phsw_delay+quant_delay  dbl_ovrd=off  reg_retiming=off  block_type=delay
  Delay2 : xbsIndex_r4/Delay  en=off  latency=2  dbl_ovrd=off  reg_retiming=off  block_type=delay
  Inverter : xbsIndex_r4/Inverter  en=off  latency=0  dbl_ovrd=off  block_type=inv
  Slice1 : xbsIndex_r4/Slice  nbits=1  boolean_output=on  mode=Lower Bit Location + Width  bit1=0  base1=MSB of Input  bit0=0  base0=LSB of Input  dbl_ovrd=off  block_type=slice
      settings: infoedit="Extracts a given range of bits from each input sample and presents it at the output.  The output type is ordinarily unsigned with binary point at zero, but can be Boolean when the slice is one bit wide.<P><P>Hardware notes: In hardware this block costs nothing."  block_version=10.1.3
  Slice9 : xbsIndex_r4/Slice  nbits=1  boolean_output=on  mode=Lower Bit Location + Width  bit1=0  base1=MSB of Input  bit0=0  base0=LSB of Input  dbl_ovrd=off  block_type=slice
      settings: infoedit="Extracts a given range of bits from each input sample and presents it at the output.  The output type is ordinarily unsigned with binary point at zero, but can be Boolean when the slice is one bit wide.<P><P>Hardware notes: In hardware this block costs nothing."  block_version=10.1.3
  Subsystem : Subsystem
  first : xbsIndex_r4/Register  init=0  rst=off  en=on  dbl_ovrd=off  block_type=register
  oob_reg : xbsIndex_r4/Register  init=0  rst=off  en=on  dbl_ovrd=off  block_type=register
  second : xbsIndex_r4/Register  init=0  rst=off  en=on  dbl_ovrd=off  block_type=register
  dout : Outport
  oob : Outport  Port=2
  valid : Outport  Port=3
  wires:
  Concat3/1 -> dout/1
  [int_1024pps] -> Delay8/1
  [int_1pps] -> Delay3/1
  [int_1024pps] -> Delay1/1
  [sync0] -> Subsystem/1(s)
  [walsh0] -> Delay5/1
  [walsh1] -> Delay4/1
  [walsh2] -> Delay7/1
  [walsh3] -> Delay6/1
  BitBasher1/1 -> oob_reg/1
  Counter/1 -> Slice1/1
  din/1 -> second/1, first/1
  Inverter/1 -> second/2
  first/1 -> Concat3/1  "first"
  second/1 -> Concat3/2  "second"
  oob_reg/1 -> oob/1  "oob"
  Delay2/1 -> valid/1  "valid"
  [start_xaui] -> Slice9/1
  Subsystem/1(ss) -> BitBasher1/3
  Delay3/1 -> BitBasher1/1
  Delay1/1 -> BitBasher1/2
  Delay5/1 -> BitBasher1/4
  Delay4/1 -> BitBasher1/5
  Delay7/1 -> BitBasher1/6
  Delay6/1 -> BitBasher1/7
  Delay8/1 -> Counter/1
  Slice9/1 -> Counter/2
  Slice1/1 -> oob_reg/2, first/2, Inverter/1, Delay2/1

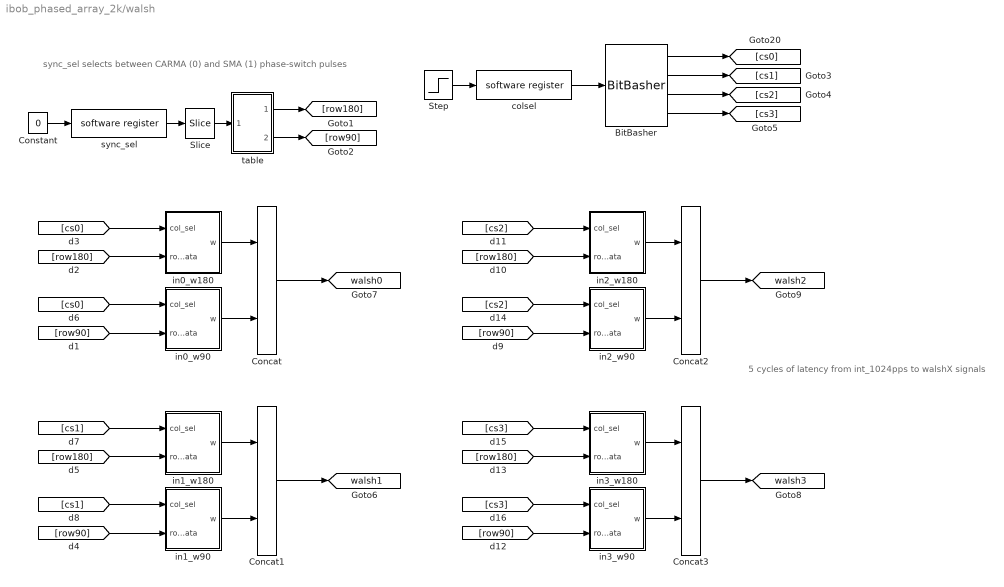
== system ibob_phased_array_2k/walsh ==
  note: 5 cycles of latency from int_1024pps to walshX signals
  note: sync_sel selects between CARMA (0) and SMA (1) phase-switch pulses
  BitBasher : xbsIndex_r4/BitBasher  bitexpr=|  display_expr=off  sr_1=1  arith_type1=Unsigned  bin_pt1=0  sr_2=2  arith_type2=Unsigned  bin_pt2=0  sr_3=3  arith_type3=Unsigned  bin_pt3=0  sr_4=4  arith_type4=Unsigned  bin_pt4=0  dbl_ovrd=off  block_type=bitbasher
      | <html><head><meta name="qrichtext" content="1" /><style type="text/css">
      | p, li { white-space: pre-wrap; }
      | </style></head><body style=" font-family:'MS Shell Dlg 2'; font-size:8.25pt; font-weight:400; font-style:normal;">
      | <p style=" margin-top:12px; margin-bottom:12px; margin-left:0px; margin-right:0px; -qt-block-indent:0; text-indent:0px; font-family:'MS Shell Dlg'; font-size:8pt;">cs0={cs[4:0]}<br />cs1={cs[12:8]}<br />cs2={cs[20:16]}<br />cs3={cs[28:24]}<br /></p></body></html>
      settings: block_version=10.1.3
  Concat{,1..3} (4 alike) : xbsIndex_r4/Concat  num_inputs=2  dbl_ovrd=off  block_type=concat
      settings: block_version=10.1.3
  Constant : Constant  Value=0  OutDataType=sfix(16)  OutScaling=2^0
  Slice : xbsIndex_r4/Slice  nbits=1  boolean_output=on  mode=Lower Bit Location + Width  bit1=0  base1=MSB of Input  bit0=0  base0=LSB of Input  dbl_ovrd=off  block_type=slice
      settings: infoedit="Extracts a given range of bits from each input sample and presents it at the output.  The output type is ordinarily unsigned with binary point at zero, but can be Boolean when the slice is one bit wide.<P><P>Hardware notes: In hardware this block costs nothing."  block_version=10.1.3
  Step : Step  Time=200  Before=1  After=0  SampleTime=1
  colsel : xps_library/software register  Tag=xps:sw_reg  SystemSampleTime=-1  io_dir=From Processor  arith_type=Unsigned  bitwidth=32  bin_pt=0  sample_period=1  gw_name=ibob_phased_array_2k_walsh_colsel_user_data_out
      link override dbe_xaui_corr_onepps_sync_arm1pps_user_data_out: arith_type=Unsigned  n_bits=32  bin_pt=0  period=1
      link override dbe_xaui_onepps_sync_arm1pps_user_data_out: arith_type=Unsigned  n_bits=32  bin_pt=0  period=1
      link override ibob_phased_array_2k_onepps_sync_arm1pps_user_data_out: arith_type=Unsigned  n_bits=32  bin_pt=0  period=1
      link override ibob_phased_array_2k_walsh_colsel_user_data_out: arith_type=Unsigned  n_bits=32  bin_pt=0  period=1
      link override vlbipfb2_m3_ibob_onepps_sync_arm1pps_user_data_out: arith_type=Unsigned  n_bits=32  bin_pt=0  period=1
      link override vlbipfb2_m3_roach_onepps_sync_arm1pps_user_data_out: arith_type=Unsigned  n_bits=32  bin_pt=0  period=1
  in0_w180 : Subsystem
  in0_w90 : Subsystem
  in1_w180 : Subsystem
  in1_w90 : Subsystem
  in2_w180 : Subsystem
  in2_w90 : Subsystem
  in3_w180 : Subsystem
  in3_w90 : Subsystem
  sync_sel : xps_library/software register  Tag=xps:sw_reg  SystemSampleTime=-1  io_dir=From Processor  arith_type=Unsigned  bitwidth=32  bin_pt=0  sample_period=1  gw_name=ibob_phased_array_2k_walsh_sync_sel_user_data_out
      link override dbe_xaui_corr_onepps_sync_arm1pps_user_data_out: arith_type=Unsigned  n_bits=32  bin_pt=0  period=1
      link override dbe_xaui_onepps_sync_arm1pps_user_data_out: arith_type=Unsigned  n_bits=32  bin_pt=0  period=1
      link override ibob_phased_array_2k_onepps_sync_arm1pps_user_data_out: arith_type=Unsigned  n_bits=32  bin_pt=0  period=1
      link override ibob_phased_array_2k_walsh_colsel_user_data_out: arith_type=Unsigned  n_bits=32  bin_pt=0  period=1
      link override ibob_phased_array_2k_walsh_sync_sel_user_data_out: arith_type=Unsigned  n_bits=32  bin_pt=0  period=1
      link override vlbipfb2_m3_ibob_onepps_sync_arm1pps_user_data_out: arith_type=Unsigned  n_bits=32  bin_pt=0  period=1
      link override vlbipfb2_m3_roach_onepps_sync_arm1pps_user_data_out: arith_type=Unsigned  n_bits=32  bin_pt=0  period=1
  table : Subsystem
  tag scope: walsh0=global, walsh1=global, walsh2=global, walsh3=global
  wires:
  Step/1 -> colsel/1
  colsel/1 -> BitBasher/1
  BitBasher/1 -> [cs0]
  BitBasher/2 -> [cs1]
  BitBasher/3 -> [cs2]
  BitBasher/4 -> [cs3]
  table/2(row90) -> [row90]
  table/1(row180) -> [row180]
  [cs0] -> in0_w90/1(col_sel)
  [row90] -> in0_w90/2(row_data)
  [cs0] -> in0_w180/1(col_sel)
  [row180] -> in0_w180/2(row_data)
  in0_w180/1(w) -> Concat/1
  Concat/1 -> [walsh0]
  in0_w90/1(w) -> Concat/2
  [cs1] -> in1_w90/1(col_sel)
  [row90] -> in1_w90/2(row_data)
  [cs1] -> in1_w180/1(col_sel)
  [row180] -> in1_w180/2(row_data)
  in1_w180/1(w) -> Concat1/1
  Concat1/1 -> [walsh1]
  in1_w90/1(w) -> Concat1/2
  [cs2] -> in2_w90/1(col_sel)
  [row90] -> in2_w90/2(row_data)
  [cs2] -> in2_w180/1(col_sel)
  [row180] -> in2_w180/2(row_data)
  in2_w180/1(w) -> Concat2/1
  Concat2/1 -> [walsh2]
  in2_w90/1(w) -> Concat2/2
  [cs3] -> in3_w90/1(col_sel)
  [row90] -> in3_w90/2(row_data)
  [cs3] -> in3_w180/1(col_sel)
  [row180] -> in3_w180/2(row_data)
  in3_w180/1(w) -> Concat3/1
  Concat3/1 -> [walsh3]
  in3_w90/1(w) -> Concat3/2
  Constant/1 -> sync_sel/1
  sync_sel/1 -> Slice/1
  Slice/1 -> table/1(sync_sel)

== system ibob_phased_array_2k/xaui0 ==
  din : Inport  OutDataType=sfix(16)  OutScaling=2^0
  oob : Inport  Port=2  OutDataType=sfix(16)  OutScaling=2^0
  valid : Inport  Port=3  OutDataType=sfix(16)  OutScaling=2^0
  Constant22 : xbsIndex_r4/Constant  arith_type=Boolean  const=0  n_bits=32  bin_pt=0  explicit_period=on  period=1  equ=P=C  opselect=C  inp2=PCIN>>17  opr=+  inp1=P  carry=CIN  dbl_ovrd=off  block_type=constant
  Constant25 : xbsIndex_r4/Constant  arith_type=Boolean  const=0  n_bits=32  bin_pt=0  explicit_period=on  period=1  equ=P=C  opselect=C  inp2=PCIN>>17  opr=+  inp1=P  carry=CIN  dbl_ovrd=off  block_type=constant
  Expression1 : xbsIndex_r4/Expression  expression=a & b  align_bp=on  en=off  latency=0  precision=Full  arith_type=Unsigned  n_bits=8  bin_pt=2  dbl_ovrd=off  block_type=expr
      settings: xl_area=[0, 0, 0, 0, 0, 0, 0]  block_version=10.1.3
  Inverter : xbsIndex_r4/Inverter  en=off  latency=0  dbl_ovrd=off  block_type=inv
      settings: xl_area=[0, 0, 0, 0, 0, 0, 0]
  Terminator{,1..3,6,8..9} (7 alike) : Terminator
  XAUI_1 : xps_library/XAUI  Tag=xps:xaui  SystemSampleTime=-1  demux=1  port=iBOB:1  open_phy=off  show_param=off  pre_emph=3  swing=800
      link override convert_tx_data: n_bits=64
      link override convert_tx_outofband: n_bits=8
      link override ibob_phased_array_2k_xaui0_XAUI_1_rx_data: n_bits=64
      link override ibob_phased_array_2k_xaui0_XAUI_1_rx_outofband: n_bits=8
      link override ibob_phased_array_2k_xaui_1_XAUI_1_rx_data: n_bits=64
      link override ibob_phased_array_2k_xaui_1_XAUI_1_rx_outofband: n_bits=8
  rx_linkdown : xps_library/software register  Tag=xps:sw_reg  SystemSampleTime=-1  io_dir=To Processor  arith_type=Unsigned  bitwidth=32  bin_pt=0  sample_period=1  gw_name=ibob_phased_array_2k_xaui0_rx_linkdown_user_data_in
      link override convert: arith_type=Unsigned  n_bits=32  bin_pt=0
  wires:
  valid/1 -> Expression1/2
  din/1 -> XAUI_1/3
  Expression1/1 -> XAUI_1/5
  oob/1 -> XAUI_1/4
  Inverter/1 -> Expression1/1
  [linkdown_0] -> Inverter/1
  Constant25/1 -> XAUI_1/2
  Constant22/1 -> XAUI_1/1
  rx_linkdown/1 -> Terminator9/1
  XAUI_1/7 -> Terminator8/1
  XAUI_1/5 -> [linkdown_0], rx_linkdown/1
  XAUI_1/4 -> Terminator6/1
  XAUI_1/3 -> Terminator2/1
  XAUI_1/2 -> Terminator/1
  XAUI_1/1 -> Terminator1/1
  XAUI_1/6 -> Terminator3/1

== system ibob_phased_array_2k/xaui1 ==
  go : Inport  OutDataType=sfix(16)  OutScaling=2^0
  oob : Inport  Port=2  OutDataType=sfix(16)  OutScaling=2^0
  din : Inport  Port=3  OutDataType=sfix(16)  OutScaling=2^0
  Constant22 : xbsIndex_r4/Constant  arith_type=Boolean  const=0  n_bits=32  bin_pt=0  explicit_period=on  period=1  equ=P=C  opselect=C  inp2=PCIN>>17  opr=+  inp1=P  carry=CIN  dbl_ovrd=off  block_type=constant
  Constant25 : xbsIndex_r4/Constant  arith_type=Boolean  const=0  n_bits=32  bin_pt=0  explicit_period=on  period=1  equ=P=C  opselect=C  inp2=PCIN>>17  opr=+  inp1=P  carry=CIN  dbl_ovrd=off  block_type=constant
  Convert : xbsIndex_r4/Convert  arith_type=Boolean  n_bits=16  bin_pt=14  quantization=Truncate  overflow=Wrap  latency=0  dbl_ovrd=off  pipeline=off  block_type=convert
      settings: block_version=10.1.3
  Counter : xbsIndex_r4/Counter  cnt_type=Free Running  cnt_to=Inf  operation=Up  start_count=0  cnt_by_val=1  arith_type=Unsigned  n_bits=1  bin_pt=0  load_pin=off  rst=off  en=off  explicit_period=on  period=1  dbl_ovrd=off  use_behavioral_HDL=off  use_rpm=off  implementation=Fabric  block_type=counter
  Inverter : xbsIndex_r4/Inverter  en=off  latency=0  dbl_ovrd=off  block_type=inv
      settings: xl_area=[0, 0, 0, 0, 0, 0, 0]
  Logical : xbsIndex_r4/Logical  logical_function=AND  inputs=3  en=off  latency=0  precision=Full  arith_type=Unsigned  n_bits=16  bin_pt=0  align_bp=on  dbl_ovrd=off  block_type=logical
  Slice1 : xbsIndex_r4/Slice  nbits=1  boolean_output=on  mode=Lower Bit Location + Width  bit1=0  base1=MSB of Input  bit0=0  base0=LSB of Input  dbl_ovrd=off  block_type=slice
      settings: infoedit="Extracts a given range of bits from each input sample and presents it at the output.  The output type is ordinarily unsigned with binary point at zero, but can be Boolean when the slice is one bit wide.<P><P>Hardware notes: In hardware this block costs nothing."  block_version=10.1.3
  Terminator{,1..3,6,8..9} (7 alike) : Terminator
  XAUI : xps_library/XAUI  Tag=xps:xaui  SystemSampleTime=-1  demux=1  port=iBOB:0  open_phy=off  show_param=off  pre_emph=3  swing=800
      link override convert_tx_data: n_bits=64
      link override convert_tx_outofband: n_bits=8
      link override ibob_phased_array_2k_xaui1_XAUI_rx_data: n_bits=64
      link override ibob_phased_array_2k_xaui1_XAUI_rx_outofband: n_bits=8
      link override ibob_phased_array_2k_xaui_0_XAUI_0_rx_data: n_bits=32
      link override ibob_phased_array_2k_xaui_0_XAUI_0_rx_outofband: n_bits=4
  din_demux2 : Subsystem
  oob_demux2 : Subsystem
  rx_linkdown : xps_library/software register  Tag=xps:sw_reg  SystemSampleTime=-1  io_dir=To Processor  arith_type=Unsigned  bitwidth=32  bin_pt=0  sample_period=1  gw_name=ibob_phased_array_2k_xaui1_rx_linkdown_user_data_in
      link override convert: arith_type=Unsigned  n_bits=32  bin_pt=0
  wires:
  XAUI/1 -> Terminator1/1
  XAUI/2 -> Terminator/1
  XAUI/3 -> Terminator2/1
  XAUI/4 -> Terminator6/1
  XAUI/5 -> [linkdown_0], rx_linkdown/1
  XAUI/7 -> Terminator8/1
  rx_linkdown/1 -> Terminator9/1
  Constant22/1 -> XAUI/1
  Constant25/1 -> XAUI/2
  [linkdown_0] -> Inverter/1
  Inverter/1 -> Logical/2
  Slice1/1 -> Logical/3
  oob/1 -> oob_demux2/1(in)
  Logical/1 -> XAUI/5
  din/1 -> din_demux2/1(in)
  go/1 -> Slice1/1
  XAUI/6 -> Terminator3/1
  din_demux2/1(out) -> XAUI/3
  oob_demux2/1(out) -> XAUI/4
  Counter/1 -> Convert/1
  Convert/1 -> Logical/1

== system ibob_phased_array_2k/adder/Subsystem ==
  a_32_in : Inport  OutDataType=sfix(16)  OutScaling=2^0
  b_32_in : Inport  Port=2  OutDataType=sfix(16)  OutScaling=2^0
  AddSub{1..4} (4 alike) : xbsIndex_r4/AddSub  mode=Addition  use_carryin=off  use_carryout=off  en=off  latency=5  precision=Full  arith_type="Signed  (2's comp)"  n_bits=9  bin_pt=6  quantization=Truncate  overflow=Wrap  dbl_ovrd=off  use_behavioral_HDL=on  pipelined=on  use_rpm=on  hw_selection=Fabric  block_type=addsub
      settings: xl_area=[0, 0, 0, 0, 0, 0, 0]  block_version=10.1.3
  BitBasher : xbsIndex_r4/BitBasher  bitexpr=|  display_expr=off  sr_1=1  arith_type1="Signed  (2's comp)"  bin_pt1=0  sr_2=2  arith_type2="Signed  (2's comp)"  bin_pt2=0  sr_3=3  arith_type3="Signed  (2's comp)"  bin_pt3=0  sr_4=4  arith_type4="Signed  (2's comp)"  bin_pt4=0  dbl_ovrd=off  block_type=bitbasher
      | <html><head><meta name="qrichtext" content="1" /><style type="text/css">
      | p, li { white-space: pre-wrap; }
      | </style></head><body style=" font-family:'MS Shell Dlg 2'; font-size:8.25pt; font-weight:400; font-style:normal;">
      | <p style=" margin-top:12px; margin-bottom:12px; margin-left:0px; margin-right:0px; -qt-block-indent:0; text-indent:0px; font-family:'MS Shell Dlg'; font-size:8pt;">a0={a[31:24]}<br />a1={a[23:16]}<br />a2={a[15:8]}<br />a3={a[7:0]}<br /></p></body></html>
      settings: block_version=10.1.3
  BitBasher1 : xbsIndex_r4/BitBasher  bitexpr=|  display_expr=off  sr_1=1  arith_type1="Signed  (2's comp)"  bin_pt1=0  sr_2=2  arith_type2="Signed  (2's comp)"  bin_pt2=0  sr_3=3  arith_type3="Signed  (2's comp)"  bin_pt3=0  sr_4=4  arith_type4="Signed  (2's comp)"  bin_pt4=0  dbl_ovrd=off  block_type=bitbasher
      | <html><head><meta name="qrichtext" content="1" /><style type="text/css">
      | p, li { white-space: pre-wrap; }
      | </style></head><body style=" font-family:'MS Shell Dlg 2'; font-size:8.25pt; font-weight:400; font-style:normal;">
      | <p style=" margin-top:12px; margin-bottom:12px; margin-left:0px; margin-right:0px; -qt-block-indent:0; text-indent:0px; font-family:'MS Shell Dlg'; font-size:8pt;">b0={b[31:24]}<br />b1={b[23:16]}<br />b2={b[15:8]}<br />b3={b[7:0]}<br /></p></body></html>
      settings: block_version=10.1.3
  BitBasher2 : xbsIndex_r4/BitBasher  bitexpr=|  display_expr=off  sr_1=1  arith_type1=Unsigned  bin_pt1=0  sr_2=2  arith_type2=Unsigned  bin_pt2=0  sr_3=3  arith_type3=Unsigned  bin_pt3=0  sr_4=4  arith_type4=Unsigned  bin_pt4=0  dbl_ovrd=off  block_type=bitbasher
      | <html><head><meta name="qrichtext" content="1" /><style type="text/css">
      | p, li { white-space: pre-wrap; }
      | </style></head><body style=" font-family:'MS Shell Dlg 2'; font-size:8.25pt; font-weight:400; font-style:normal;">
      | <p style=" margin-top:12px; margin-bottom:12px; margin-left:0px; margin-right:0px; -qt-block-indent:0; text-indent:0px; font-family:'MS Shell Dlg'; font-size:8pt;">c={c0,c1,c2,c3}</p></body></html>
      settings: block_version=10.1.3
  Out1 : Outport  OutDataType=sfix(16)  OutScaling=2^0
  wires:
  BitBasher1/4 -> AddSub4/2
  BitBasher1/3 -> AddSub3/2
  BitBasher1/2 -> AddSub2/2
  BitBasher1/1 -> AddSub1/2
  BitBasher/4 -> AddSub4/1
  BitBasher/3 -> AddSub3/1
  BitBasher/2 -> AddSub2/1
  BitBasher/1 -> AddSub1/1
  a_32_in/1 -> BitBasher/1
  b_32_in/1 -> BitBasher1/1
  AddSub1/1 -> BitBasher2/1
  AddSub2/1 -> BitBasher2/2
  AddSub3/1 -> BitBasher2/3
  AddSub4/1 -> BitBasher2/4
  BitBasher2/1 -> Out1/1
